simulink model "record_plant"  (R2025a)
settings: Solver=FixedStepAuto  StartTime=0.0  StopTime=Inf  RelTol=1e-3  EnableMultiTasking=on
libraries: arduinolib x3, arduinosensorlib x1
settings Model: SimulationMode=external  SILPILModeSetting=veronly  ExtModeTrigDuration=2  Creator=AthaariqRamadhani  LastModifiedBy=Athaariq
settings SolverCC: AutoInsertRateTranBlk=on
settings OptimizationCC: EnhancedBackFolding=on  PassReuseOutputArgsAs=Individual arguments  ZeroExternalMemoryAtStartup=off  ZeroInternalMemoryAtStartup=off  MaxStackSize=64  OptimizeBlockOrder=speed  DifferentSizesBufferReuse=on  EfficientTunableParamExpr=on
settings DebuggingCC: ParameterTunabilityLossMsg=error
settings HardwareCC: ProdBitPerInt=16.0  ProdBitPerPointer=16.0  ProdBitPerSizeT=16.0  ProdBitPerPtrDiffT=16.0  ProdLargestAtomicFloat=None  ProdWordSize=8.0  ProdHWDeviceType=Atmel->AVR
settings SFSimCC: MATLABDynamicMemAlloc=off
settings RTWCC: SystemTargetFile=ert.tlc  HardwareBoard=Arduino Uno  TemplateMakefile=ert_default_tmf  Toolchain=Arduino AVR  BuildConfiguration=Faster Runs  Description=Embedded Coder
settings CodeAppCC: ForceParamTrailComments=on  IgnoreCustomStorageClasses=off  OperatorAnnotations=on  SimulinkDataObjDesc=on  SFDataObjDesc=on  InsertBlockDesc=on
settings ERTTargetCC: ExtModeTransport=3.0  ExtModeAutomaticAllocSize=off  ExtModeStaticAllocSize=250.0  InlinedParameterPlacement=Hierarchical  SupportContinuousTime=on  SupportVariableSizeSignals=on

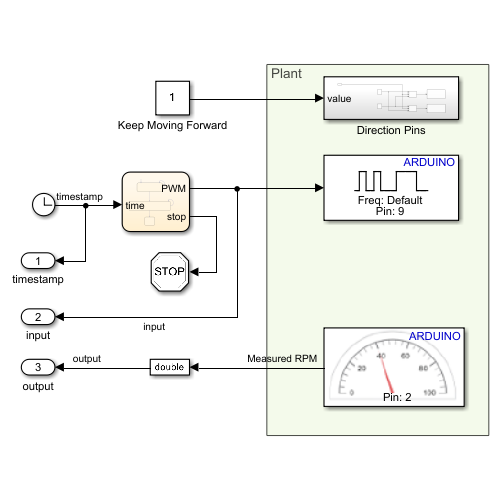
[thumbnail: Simulink's stored preview of the top-level diagram]
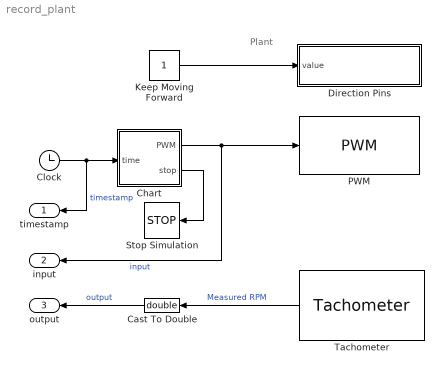
== system record_plant ==
  note: Plant
  Cast To Double : DataTypeConversion  OutDataTypeStr=double  SaturateOnIntegerOverflow=off  RndMeth=Floor
  Chart : Stateflow chart  TreatAsAtomicUnit=on
  Clock : Clock
  Direction Pins : Subsystem
  Keep Moving Forward : Constant
  PWM : arduinolib/PWM  pinNumber=9  frequencyType=Default  desiredFrequency=490.2  achievableFrequency=490.2
  Stop Simulation : Stop
  Tachometer : arduinosensorlib/Tachometer  PinNumber=2  InterruptMode=RISING  PulseCountperRotation=20  SampleTime=0.1  blockPlatform=ARDUINO
  timestamp : Outport
  input : Outport  Port=2
  output : Outport  Port=3
  wires:
  Keep Moving Forward/1 -> Direction Pins/1(value)
  Tachometer/1 -> Cast To Double/1  "Measured RPM"
  Chart/1(PWM) -> input/1, PWM/1  "input"
  Cast To Double/1 -> output/1  "output"
  Clock/1 -> timestamp/1, Chart/1(time)  "timestamp"
  Chart/2(stop) -> Stop Simulation/1

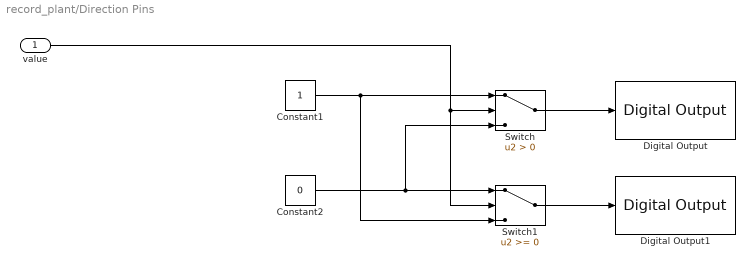
== system record_plant/Direction Pins ==
  value : Inport
  Constant1 : Constant
  Constant2 : Constant  Value=0
  Digital Output : arduinolib/Digital Output  pinNumber=3  Direction=output  blockPlatform=arduino
  Digital Output1 : arduinolib/Digital Output  pinNumber=6  Direction=output  blockPlatform=arduino
  Switch : Switch  Criteria=u2 > Threshold  SaturateOnIntegerOverflow=off  InputSameDT=off
  Switch1 : Switch  SaturateOnIntegerOverflow=off  InputSameDT=off
  wires:
  Constant2/1 -> Switch/3, Switch1/1
  Switch1/1 -> Digital Output1/1
  value/1 -> Switch1/2, Switch/2
  Constant1/1 -> Switch1/3, Switch/1
  Switch/1 -> Digital Output/1

== stateflow chart record_plant/Chart ==
  state Accelerating
    step = floor(time / interval);
    PWM = step * increment;
  state Deaccelerating
    step = floor((time - deaccelerate_start) / interval);
    PWM = 255 - (step * increment);
  state Stop
    PWM = 0;
    stop = true;
  (default) -> Accelerating
  Accelerating -> Accelerating [order 1] : [PWM <= 255]
  Accelerating -> Deaccelerating [order 2] : [PWM > 255]{deaccelerate_start = time;}
  Deaccelerating -> Deaccelerating [order 1] : [PWM >= 0]
  Deaccelerating -> Stop [order 2] : [PWM < 0]
  data: time input; step local =0; interval constant double =5; PWM output =0; stop output boolean =false; increment constant double =10; deaccelerate_start local =0
